simulink model "diffContGazebo"  (R2022b)
settings: Solver=FixedStepAuto  StartTime=0.0  StopTime=inf  FixedStep=Ts  RelTol=1e-3
PreLoadFcn:
  | Ts = 0.1;
undefined symbols (not defined in the file or in its folder): angular, linear
libraries: ros2lib x3
settings Model: Creator=System-10  LastModifiedBy=System-10

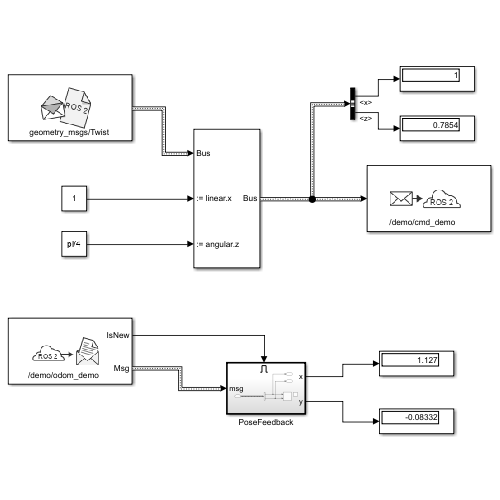
[thumbnail: Simulink's stored preview of the top-level diagram]
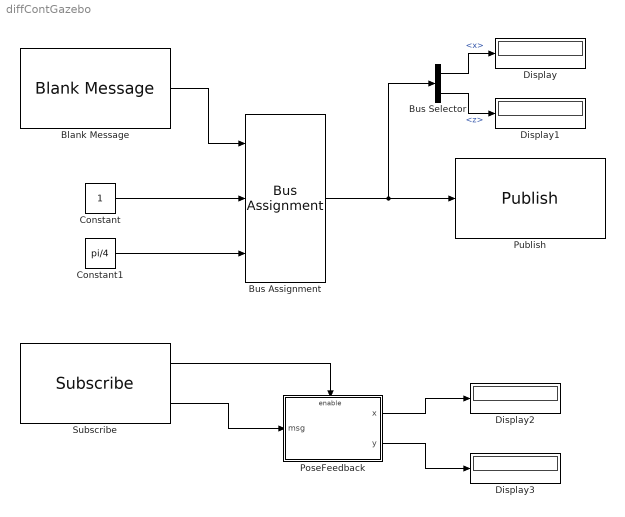
== system diffContGazebo ==
  Blank Message : ros2lib/Blank Message  messageClass=Message  entityType=geometry_msgs/Twist  messageType=geometry_msgs/Twist  SampleTime=Ts
      settings: LibrarySourceBlock=roslib/ROS 2/Blank Message
  Bus Assignment : BusAssignment  AssignedSignals=linear.x,angular.z
  Bus Selector : BusSelector  OutputSignals=linear.x,angular.z
  Constant : Constant  VectorParams1D=off  SampleTime=Ts
  Constant1 : Constant  Value=pi/4  SampleTime=Ts
  Display{,1..3} (4 alike) : Display
  PoseFeedback : Subsystem
  Publish : ros2lib/Publish  topicSource=Specify your own  topic=/demo/cmd_demo  messageType=geometry_msgs/Twist  QOSHistory=Keep last  QOSDepth=1  QOSReliability=Reliable  QOSDurability=Volatile
      settings: LibrarySourceBlock=roslib/ROS 2/Publish
  Subscribe : ros2lib/Subscribe  topicSource=Specify your own  topic=/demo/odom_demo  messageType=nav_msgs/Odometry  sampleTime=Ts  QOSHistory=Keep last  QOSDepth=1  QOSReliability=Reliable  QOSDurability=Volatile
      settings: LibrarySourceBlock=roslib/ROS 2/Subscribe
  wires:
  Blank Message/1 -> Bus Assignment/1
  Bus Assignment/1 -> Publish/1, Bus Selector/1
  Constant/1 -> Bus Assignment/2
  Constant1/1 -> Bus Assignment/3
  Bus Selector/1 -> Display/1  "<x>"
  Bus Selector/2 -> Display1/1  "<z>"
  Subscribe/2 -> PoseFeedback/1(msg)
  Subscribe/1 -> PoseFeedback/Enable
  PoseFeedback/1(x) -> Display2/1
  PoseFeedback/2(y) -> Display3/1

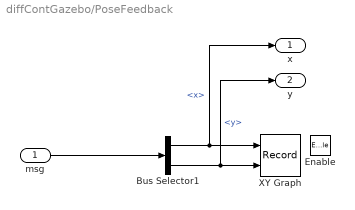
== system diffContGazebo/PoseFeedback ==
  msg : Inport
  Enable : EnablePort
  Bus Selector1 : BusSelector  OutputSignals=pose.pose.position.x,pose.pose.position.y
  XY Graph : Record  FileSettingsInternal="{\"entries\":[{\"content\":{\"excelSettings\":{\"content\":{},\"type\":\"Streamout.ExcelSettings\"}},\"type\":\"Streamout.FileSettingStorage\",\"uuid\":\"8e07aba7-d6b7-4f3d-95c1-9b04d42fe51c\"}],\"packageUris\":[\"http://schema.mathworks.com/mf0/streamout_blocks/R2020a\"],\"version\":\"1.0\"}"  Layout=[1 1]  SignalsInternal="{\"entries\":[{\"content\":{\"signals\":[{\"content\":{\"blockPath\":[\"diffContGazebo/PoseFeedback/XY Graph\"],\"channel\":[],\"dimensions\":[1],\"domain\":\"diffContGazebo/PoseFeedback/XY Graph\",\"lineColor\":\"#a2142f\",\"plots\":[1],\"port\":1,\"sid\":[\"\"],\"signalID\":375,\"signalName\":\"<x>\"},\"type\":\"RecordBlkView.Signal\",\"uuid\":\"0e74358a-b4c8-426c-9d2c-fa4a2ca85053\"},{\"content\":{\"blockPath\":[\"diffContGazebo/PoseFeedback/XY Graph\"],\"channel\":[],\"dimensions\":[1],\"domain\":\"diffContGazebo/PoseFeedback/XY Graph\",\"lineColor\":\"#139fff\",\"plots\":[1],\"port\":2,\"sid\":[\"\"],\"signalID\":379,\"signalName\":\"<y>\"},\"type\":\"RecordBlkView.Signal\",\"uuid\":\"df9b493f-ba8b-471d-9638-13e81596006c\"}]},\"type\":\"RecordBlkView.InputSignals\",\"uuid\":\"08bcb471-31d0-4c59-b5b4-fffedc929894\"}],\"packageUris\":[\"http://schema.mathworks.com/mf0/streamout_blocks/R2020a\"],\"version\":\"1.0\"}"  VisualizationBindings="{\"xyplotplugin\":{\"info\":[{\"series\":[{\"bindingParametersList\":[{\"parameter\":\"X-Axis\",\"signalID\":375,\"signalName\":\"<x>\"},{\"parameter\":\"Y-Axis\",\"signalID\":379,\"signalName\":\"<y>\"}],\"seriesID\":3202}],\"subplotID\":1}]}}"  CompatibilityTag=XY
  x : Outport
  y : Outport  Port=2
  wires:
  msg/1 -> Bus Selector1/1
  Bus Selector1/1 -> XY Graph/1, x/1  "<x>"
  Bus Selector1/2 -> XY Graph/2, y/1  "<y>"
